simulink model "SimpleReverb"  (R2020a)
settings: Solver=VariableStepAuto  StartTime=0.0  StopTime=100000  RelTol=1e-3
libraries: audiosources x1, dspsnks4 x1, dspsrcs4 x1
settings Model: Creator=ace  LastModifiedBy=ace

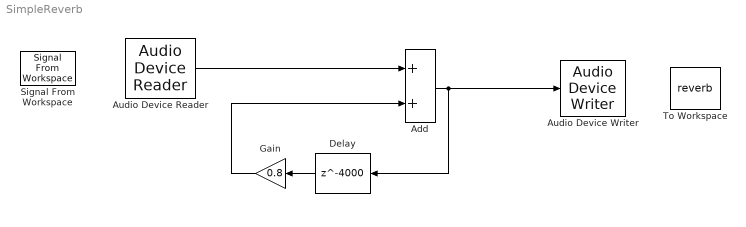
== system SimpleReverb ==
  Add : Sum
  Audio Device Reader : audiosources/Audio Device Reader  Driver=CoreAudio  Device=Default  SampleRate=44100  NumChannels=1  SamplesPerFrame=1024  BitDepth=16-bit integer  NumBuffers=10  DefaultInputChannelMapping=on  InputChannelMapping=1:2  OutputNumOverrunSamples=off  OutputDataType=double  DriverIdx=5  DeviceWarnFlag=''
      settings: SourceProductBaseCode=AU
  Audio Device Writer : dspsnks4/Audio Device Writer  Driver=CoreAudio  Device=Default  InheritSampleRate=on  SampleRate=44100  BitDepth=16-bit integer  BufferSize=4096  NumBuffers=10  DefaultOutputChannelMapping=on  OutputChannelMapping=1:2  OutputNumUnderrunSamples=off  DriverIdx=5  DeviceWarnFlag=''
  Delay : Delay  DelayLength=4000  InputProcessing=Columns as channels (frame based)
  Gain : Gain  Gain=0.8
  Signal From Workspace : dspsrcs4/Signal From Workspace  X=Hello  Ts=1  nsamps=1  OutputAfterFinalValue=Setting to zero  ignoreOrWarnInputAndFrameLengths=off  OutputFrames=off
  To Workspace : ToWorkspace  VariableName=reverb  SampleTime=-1
      settings: Save2DSignal=2-D array (concatenate along first dimension)
  wires:
  Add/1 -> Delay/1, Audio Device Writer/1
  Gain/1 -> Add/2
  Delay/1 -> Gain/1
  Audio Device Reader/1 -> Add/1
